simulink model "risingDebounce_th"  (R2018b)
settings: Solver=FixedStepAuto  StartTime=0.0  StopTime=10.0  FixedStep=0.01  RelTol=1e-3
libraries: imageProcessingFault_ul x1
settings Model: Creator=mcobb  LastModifiedBy=mcobb

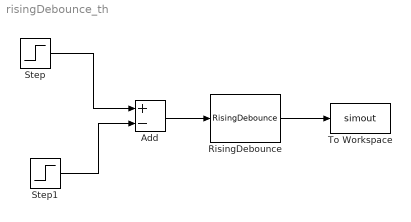
== system risingDebounce_th ==
  Add : Sum  Inputs=+-
  RisingDebounce : imageProcessingFault_ul/RisingDebounce  threshold=0.5  timeDelay_s=1
  Step : Step  SampleTime=0
  Step1 : Step  Time=3  SampleTime=0
  To Workspace : ToWorkspace  VariableName=simout  SaveFormat=Timeseries  SampleTime=-1
  wires:
  RisingDebounce/1 -> To Workspace/1
  Add/1 -> RisingDebounce/1
  Step/1 -> Add/1
  Step1/1 -> Add/2
